simulink model "ackerman_ROS_controller_neuro_2022_v2"  (R2024b)
settings: Solver=FixedStepDiscrete  StartTime=0.0  StopTime=200  FixedStep=0.1  RelTol=1e-3
undefined symbols (not defined in the file or in its folder): Angular, Linear
libraries: neural x58, robotlib x15, robotcorelib x1
(part 2 of 2)

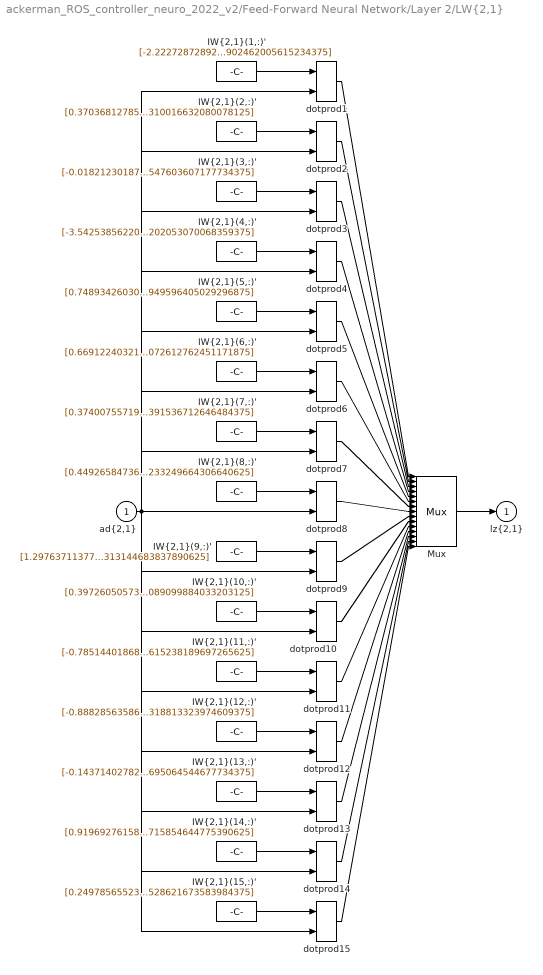
== system ackerman_ROS_controller_neuro_2022_v2/Feed-Forward Neural Network/Layer 2/LW{2,1} ==
  "ad{2,1}" : Inport  PortDimensions=30  SampleTime=0.1
      mask Display: e = 0.06;c1 = [120 230 180]/255;c2 = ([120 230 180]+0)/(256+128);c3 = ([120 230 180]+128)/(256+128);patch([0 1 1 0],[0 0 1 1],c1);patch([0 1 1 1-e 1-e 0+e],[0 0 1 1-e 0+e 0+e],c2);patch([0 0 1 1-e 0+e 0+e],[0 1 1 1-e 1-e 0+e],c3);plot([0 1 1 0 0],[0 0 1 1 0]);
  "IW{2,1}(1,:)'" : Constant  Value=[-2.222728728926282482092346981517039239406585693359375;-0.2105279558412855578364286657233606092631816864013671875;-0.172396838156845644274284268249175511300563812255859375;0.390555860841058477550546967904665507376194000244140625;0.29166384292928881905027083121240139007568359375;-0.52956405558462293914345764278550632297992706298828125;-0.2387539511607948694571490477756015025079250335693359375;-2.3297673734605712780876274337060749530792236328125;-1.0301886589615254496976604059454984962940216064453125;-0.8572014533549923154254202017909847199916839599609375;-0.96740765287111474268755273442366160452365875244140625;0.90630995398566727150324595640995539724826812744140625;-0.42554772872272794703718545861192978918552398681640625;-1.060064209881802721469057360081933438777923583984375;-0.135197213909062252668036308023147284984588623046875;0.230054241181365692892057950302842073142528533935546875;-0.827824536526168497374555954593233764171600341796875;-1.276066373600390324583031542715616524219512939453125;-0.58840911579547860998928854314726777374744415283203125;0.35688786142330453099447140630218200385570526123046875;0.795085260758974232686568939243443310260772705078125;-2.268416885537336558087417870410718023777008056640625;0.61193976284335882542819717855309136211872100830078125;1.7425116564191933665739497882896102964878082275390625;0.11927294085530919243165470788881066255271434783935546875;-0.2109230753914088374312285623091156594455242156982421875;-1.819948975500169208174838786362670361995697021484375;1.3342711728381899671802557350019924342632293701171875;1.172678912458624100878523677238263189792633056640625;-0.411449480689598467986201058010919950902462005615234375]
      mask Display: e = 0.06;c1 = [120 150 230]/255;c2 = ([120 150 230]+0)/383;c3 = ([120 150 230]+128)/383;patch([0 1 1 0],[0 0 1 1],c1);patch([0 1 1 1-e 1-e 0+e],[0 0 1 1-e 0+e 0+e],c2);patch([0 0 1 1-e 0+e 0+e],[0 1 1 1-e 1-e 0+e],c3);plot([0 1 1 0 0],[0 0 1 1 0]);disp('weights');
  "IW{2,1}(10,:)'" : Constant  Value=[0.397260505736018121325514584896154701709747314453125;-0.50051569273377294333471354548237286508083343505859375;0.02758078036917484265888589334281277842819690704345703125;0.383440619053087738965501785060041584074497222900390625;0.0314483306075712676364020126129616983234882354736328125;0.89079094780964995781147308662184514105319976806640625;-0.3737922284921084692399517734884284436702728271484375;-0.2002468106304216011182006695889867842197418212890625;0.4602876671052265056260921483044512569904327392578125;0.300424473405391356806148905889131128787994384765625;0.1539216720517649072963450862516765482723712921142578125;0.27531316556655927030305974767543375492095947265625;-1.317788466887037213126632195780985057353973388671875;-0.25114389862770158945437515285448171198368072509765625;-0.024189059746283221585816392007473041303455829620361328125;-0.2408523864701219707740165176801383495330810546875;0.08168961019016017510718796756918891333043575286865234375;-0.08534930377349826680077882201658212579786777496337890625;0.405079373978569190484222417580895125865936279296875;-3.302395281601825605122257911716587841510772705078125;-0.289408974864118817560409979705582372844219207763671875;-0.5678096913294385927883922704495489597320556640625;0.65866437262387267370655763443210162222385406494140625;-0.61601410378164789261035139134037308394908905029296875;0.1337985101975235624482962748516001738607883453369140625;-0.442241434107712050316507657043985091149806976318359375;1.4648271622279427361945636221207678318023681640625;-0.74575093210429244106052237839321605861186981201171875;-0.325176543537462225952339167633908800780773162841796875;0.47945924442098697415559627188486047089099884033203125]
      mask Display: e = 0.06;c1 = [120 150 230]/255;c2 = ([120 150 230]+0)/383;c3 = ([120 150 230]+128)/383;patch([0 1 1 0],[0 0 1 1],c1);patch([0 1 1 1-e 1-e 0+e],[0 0 1 1-e 0+e 0+e],c2);patch([0 0 1 1-e 0+e 0+e],[0 1 1 1-e 1-e 0+e],c3);plot([0 1 1 0 0],[0 0 1 1 0]);disp('weights');
  "IW{2,1}(11,:)'" : Constant  Value=[-0.7851440186858449354900812977575697004795074462890625;-0.40208723330404050333442000919603742659091949462890625;0.70730003574929212195598893231363035738468170166015625;-0.065367184060295902003900891941157169640064239501953125;-4.2920405936075400887830255669541656970977783203125;-0.523445857646462453516278401366434991359710693359375;-0.029332229217134374310571587329832254908978939056396484375;-0.171317200281045689536085774307139217853546142578125;-0.27023493407209941974400635444908402860164642333984375;-1.6651118212079636382583203157992102205753326416015625;-0.264468105797145025537275841998052783310413360595703125;0.277586538506012170390846449663513340055942535400390625;-0.03697520577241696082548827462233020924031734466552734375;-0.086749109060326456965839270196738652884960174560546875;-0.5897102236852784784559844410978257656097412109375;0.860204401837508125794329316704533994197845458984375;3.52278173836524644002565764822065830230712890625;-3.404212909954015042757191622513346374034881591796875;-2.895449655572719382945479082991369068622589111328125;-1.9360634251116242143808676701155491173267364501953125;1.0168561706644438924485029929201118648052215576171875;1.5208740618630673946398701446014456450939178466796875;1.18377350921994572985340710147283971309661865234375;0.257753028254375793348884826627909205853939056396484375;1.3769223840811586345722616897546686232089996337890625;-0.2545354697793398290883715162635780870914459228515625;0.154239895895388612334642175483168102800846099853515625;-0.435963640834392152090259742180933244526386260986328125;0.72813713755268627547678761402494274079799652099609375;0.66551241615256151451518462636158801615238189697265625]
      mask Display: e = 0.06;c1 = [120 150 230]/255;c2 = ([120 150 230]+0)/383;c3 = ([120 150 230]+128)/383;patch([0 1 1 0],[0 0 1 1],c1);patch([0 1 1 1-e 1-e 0+e],[0 0 1 1-e 0+e 0+e],c2);patch([0 0 1 1-e 0+e 0+e],[0 1 1 1-e 1-e 0+e],c3);plot([0 1 1 0 0],[0 0 1 1 0]);disp('weights');
  "IW{2,1}(12,:)'" : Constant  Value=[-0.88828563586649111893933650208055041730403900146484375;-0.6287976390637479706668955259374342858791351318359375;0.140039962452482902310890722219482995569705963134765625;0.34178216493342272741529086488299071788787841796875;0.06889275826908593247654977176352986134588718414306640625;-2.720725732529100771017738225054927170276641845703125;-1.1686144782811760389762412160052917897701263427734375;-0.04765305455937184075931867255349061451852321624755859375;0.1892635702445351342237955805103410966694355010986328125;-0.337729970142503777008613496946054510772228240966796875;0.26819643917410329603256968766800127923488616943359375;-0.073970398171442852675028234443743713200092315673828125;0.67889553499922550283685040994896553456783294677734375;0.2277097388882860229397664397765765897929668426513671875;0.17970819867203224884377732450957410037517547607421875;3.38343871560046860480497343814931809902191162109375;0.0859002580832470552518742579195532016456127166748046875;-0.365418601907997409039552394460770301520824432373046875;0.57476314636036018868026076233945786952972412109375;3.5484404227567569733992058900184929370880126953125;1.728437779847022515156140798353590071201324462890625;-0.855695122888823878071207218454219400882720947265625;1.677341944427493292124609070015139877796173095703125;0.1865942059121843410451901945634745061397552490234375;0.92489997299214277148848850629292428493499755859375;-0.64739057139335931534418477895087562501430511474609375;-1.596020893984157584810645857942290604114532470703125;0.94338078668932912052014216897077858448028564453125;1.0906949421572011971193205681629478931427001953125;-0.83878359303965088766830149324960075318813323974609375]
      mask Display: e = 0.06;c1 = [120 150 230]/255;c2 = ([120 150 230]+0)/383;c3 = ([120 150 230]+128)/383;patch([0 1 1 0],[0 0 1 1],c1);patch([0 1 1 1-e 1-e 0+e],[0 0 1 1-e 0+e 0+e],c2);patch([0 0 1 1-e 0+e 0+e],[0 1 1 1-e 1-e 0+e],c3);plot([0 1 1 0 0],[0 0 1 1 0]);disp('weights');
  "IW{2,1}(13,:)'" : Constant  Value=[-0.143714027822973544612494833927485160529613494873046875;0.44915448478707187263125888421200215816497802734375;0.376342062861311277277565068288822658360004425048828125;0.2972881796216662042553480205242522060871124267578125;-0.262879525804558422663603778346441686153411865234375;0.669912040415586940156345008290372788906097412109375;0.55179800426891001396967340042465366423130035400390625;-0.1280188538305278289630706467505660839378833770751953125;-0.26870732789751361480057312292046844959259033203125;-0.88992954257796819117487530093058012425899505615234375;0.10084960208333006159708844506894820369780063629150390625;-0.135564623109469206685417930202675051987171173095703125;0.05726056048422868693936749195927404798567295074462890625;-0.69087484836309298597001316011301241815090179443359375;-0.364074919202029223530558965649106539785861968994140625;-0.68698815425119785782470671620103530585765838623046875;-0.2989794608073983450680088935769163072109222412109375;-0.2292420658214328887947175417139078490436077117919921875;-0.45694834929996697159282348366104997694492340087890625;0.057371376318434579022476071941127884201705455780029296875;-0.00556462694212314819275366772899360512383282184600830078125;0.7850567827472574311542530267615802586078643798828125;0.25807628646158031759938467075699009001255035400390625;-0.219895909726642690973363869488821364939212799072265625;-1.6058331677712154306192360309069044888019561767578125;0.297515994915471593262878968744189478456974029541015625;-0.13003496096245992230677757106604985892772674560546875;-0.32177689840712420110691027730354107916355133056640625;0.0766703441941760377442705021167057566344738006591796875;0.68248575195410177141042140647186897695064544677734375]
      mask Display: e = 0.06;c1 = [120 150 230]/255;c2 = ([120 150 230]+0)/383;c3 = ([120 150 230]+128)/383;patch([0 1 1 0],[0 0 1 1],c1);patch([0 1 1 1-e 1-e 0+e],[0 0 1 1-e 0+e 0+e],c2);patch([0 0 1 1-e 0+e 0+e],[0 1 1 1-e 1-e 0+e],c3);plot([0 1 1 0 0],[0 0 1 1 0]);disp('weights');
  "IW{2,1}(14,:)'" : Constant  Value=[0.91969276158981216884313880655099637806415557861328125;0.01449508507313798134907845138741322443820536136627197265625;-0.024841524328765525464479679840223980136215686798095703125;0.475942644087020527710052419934072531759738922119140625;-0.66794373102359194671606701376731507480144500732421875;0.21243174640298911892699607051326893270015716552734375;-0.060849636143924780429248500013272860087454319000244140625;0.288282346155616375771302273278706707060337066650390625;0.280732424646566947057380048136110417544841766357421875;0.2220524545058630561111812085073324851691722869873046875;0.2369034334743520542332362310844473540782928466796875;-0.03729924671213581677253756652135052718222141265869140625;1.0143682463285033090727438320755027234554290771484375;-0.7815859333193930780225855414755642414093017578125;0.57258736722684455688892057878547348082065582275390625;0.35814399580322364702311688233749009668827056884765625;0.64259443013373529485221524737426079809665679931640625;-0.68301410998834699572768158759572543203830718994140625;-0.63194693767695875319390097502036951482295989990234375;-0.2370940255283547626330431512542418204247951507568359375;-0.328446483524902743678097749580047093331813812255859375;0.4236807135574398586186362081207334995269775390625;0.09468149668269500163209073662073933519423007965087890625;0.54508401115510152212806360694230534136295318603515625;0.4329377453036225009697091081761755049228668212890625;0.2318409242532646075130031704247812740504741668701171875;-0.07788041732279683826423166692620725370943546295166015625;1.732288734516942430019526000251062214374542236328125;-0.62127850580790855428148233841056935489177703857421875;-0.08755901720081916972393543119324021972715854644775390625]
      mask Display: e = 0.06;c1 = [120 150 230]/255;c2 = ([120 150 230]+0)/383;c3 = ([120 150 230]+128)/383;patch([0 1 1 0],[0 0 1 1],c1);patch([0 1 1 1-e 1-e 0+e],[0 0 1 1-e 0+e 0+e],c2);patch([0 0 1 1-e 0+e 0+e],[0 1 1 1-e 1-e 0+e],c3);plot([0 1 1 0 0],[0 0 1 1 0]);disp('weights');
  "IW{2,1}(15,:)'" : Constant  Value=[0.249785655239535053784294404977117665112018585205078125;0.73847329316424270562180254273698665201663970947265625;0.465590157117974523526271468654158525168895721435546875;-1.4664444230598145946231625202926807105541229248046875;0.09552762587386252890464533038539229892194271087646484375;-0.68536312255041187402326841038302518427371978759765625;-1.154815920318017941070820597815327346324920654296875;-0.323928699724852220409587744143209420144557952880859375;-0.370249587866944562808413365928572602570056915283203125;0.0389325824217096327917175813126959837973117828369140625;-1.993732515225736801056655167485587298870086669921875;0.04113107734049718799962391813096473924815654754638671875;-0.262819013803644363491684998734854161739349365234375;-0.473812061061643863268955101375468075275421142578125;0.132618304135100173457573191626579500734806060791015625;-1.1334068367848046943180406742612831294536590576171875;-0.6135879731176652196467102839960716664791107177734375;0.2134956515440565028018937709930469281971454620361328125;-0.1658605608926594088270434212972759269177913665771484375;-0.97371264213567132461690789568820036947727203369140625;-0.07709796244982607127393947621385450474917888641357421875;0.68597352663209665291077499205130152404308319091796875;-0.358154116190059712554472071133204735815525054931640625;0.159281117085610268713224968450958840548992156982421875;-0.2111179695429933611539041748983436264097690582275390625;0.45696544949359474419026128089171834290027618408203125;-0.757966704596435558727307579829357564449310302734375;-0.5657492883728132415654954456840641796588897705078125;-0.72239652871486137453160836230381391942501068115234375;-0.79745618550237595822949288049130700528621673583984375]
      mask Display: e = 0.06;c1 = [120 150 230]/255;c2 = ([120 150 230]+0)/383;c3 = ([120 150 230]+128)/383;patch([0 1 1 0],[0 0 1 1],c1);patch([0 1 1 1-e 1-e 0+e],[0 0 1 1-e 0+e 0+e],c2);patch([0 0 1 1-e 0+e 0+e],[0 1 1 1-e 1-e 0+e],c3);plot([0 1 1 0 0],[0 0 1 1 0]);disp('weights');
  "IW{2,1}(2,:)'" : Constant  Value=[0.37036812785328787622773916154983453452587127685546875;0.2372351393039373868010244450488244183361530303955078125;-0.08208151238239615177239016929888748563826084136962890625;-0.756141526114650464052147071924991905689239501953125;2.0086812621638596709772173198871314525604248046875;0.1690215724509795958141467053792439401149749755859375;-0.407657496635374538840324021293781697750091552734375;-0.3095937052135770972682848878321237862110137939453125;0.195510129566937196354814432197599671781063079833984375;0.5037980330495239744692526073777116835117340087890625;0.443237905161040168788844084701850078999996185302734375;-0.490943066941660510860145905098761431872844696044921875;0.70589503611337622857035967172123491764068603515625;-0.8529065119141279183168080635368824005126953125;0.055669596706750264225593838318673078902065753936767578125;0.625338821924220411574424360878765583038330078125;-1.087989422027583419350094118271954357624053955078125;1.07158158947521808812552990275435149669647216796875;1.48611353906423016013604865293018519878387451171875;0.958090545814744842800791957415640354156494140625;-0.2323317667295948518724202358498587273061275482177734375;-1.346824753200186020052342428243719041347503662109375;-0.4751862921685303664531829781481064856052398681640625;0.5088422892649340223414355932618491351604461669921875;0.94146787964793243741468131702276878058910369873046875;0.138924248447489073754468336119316518306732177734375;-0.2055196930009268729833138422691263258457183837890625;-1.209963306279714156943327907356433570384979248046875;-0.6989560104743810509120294227614067494869232177734375;0.17232859067709249689670514271710999310016632080078125]
      mask Display: e = 0.06;c1 = [120 150 230]/255;c2 = ([120 150 230]+0)/383;c3 = ([120 150 230]+128)/383;patch([0 1 1 0],[0 0 1 1],c1);patch([0 1 1 1-e 1-e 0+e],[0 0 1 1-e 0+e 0+e],c2);patch([0 0 1 1-e 0+e 0+e],[0 1 1 1-e 1-e 0+e],c3);plot([0 1 1 0 0],[0 0 1 1 0]);disp('weights');
  "IW{2,1}(3,:)'" : Constant  Value=[-0.0182123018709974167361753671912083518691360950469970703125;0.024485940403517043872927416714446735568344593048095703125;0.2128298437880238314079406336531974375247955322265625;-0.051489579338525791329939096385714947246015071868896484375;-0.31852585166436975239179218988283537328243255615234375;0.206244344898872056237593142213881947100162506103515625;-0.400235552853889287039379496491164900362491607666015625;0.3591282928342776070707031976780854165554046630859375;-0.08424416730005150621973797342434409074485301971435546875;0.58898108879171007234987200718023814260959625244140625;-0.29721325209900217867442506758379749953746795654296875;-0.362388635788180979435679773814626969397068023681640625;-0.329638246275588964184777296395623125135898590087890625;0.226923828148602513277154457682627253234386444091796875;-0.483766509869606731175650793375098146498203277587890625;0.19172010346523549184638568476657383143901824951171875;-0.0263940785096612971771801170461912988685071468353271484375;-0.0005120153139836400822682005440356078906916081905364990234375;-1.0270891419762746554766863482655026018619537353515625;0.1059209548060698613536345646934933029115200042724609375;-0.4764076619161372594390968515654094517230987548828125;-0.329461204090122639076554378334549255669116973876953125;-0.11978287653907686294285639405643451027572154998779296875;0.411122448073615365249366959687904454767704010009765625;0.130648242560915506249585860132356174290180206298828125;-0.076200560206313994182636406549136154353618621826171875;-0.007143702287312325878432250902960731764324009418487548828125;-0.409182084200852280719828968358342535793781280517578125;0.3603122929486672898491406158427707850933074951171875;-0.313453816588288469713319273068918846547603607177734375]
      mask Display: e = 0.06;c1 = [120 150 230]/255;c2 = ([120 150 230]+0)/383;c3 = ([120 150 230]+128)/383;patch([0 1 1 0],[0 0 1 1],c1);patch([0 1 1 1-e 1-e 0+e],[0 0 1 1-e 0+e 0+e],c2);patch([0 0 1 1-e 0+e 0+e],[0 1 1 1-e 1-e 0+e],c3);plot([0 1 1 0 0],[0 0 1 1 0]);disp('weights');
  "IW{2,1}(4,:)'" : Constant  Value=[-3.5425385622002547592046539648436009883880615234375;0.4922999974317985305560796405188739299774169921875;0.56569220858917323990766590213752351701259613037109375;0.25133938159345758922569302740157581865787506103515625;1.87960059681972069256516988389194011688232421875;-1.12608026029798935496728518046438694000244140625;-1.6290518269770715154010076730628497898578643798828125;-0.433087998011002561771221053277258761227130889892578125;1.1179898320468755201773092267103493213653564453125;3.37981348955477667317381929024122655391693115234375;-0.1173248613884605717760933885074337013065814971923828125;-0.91395205660366241051661972960573621094226837158203125;-0.97563873657677679940292136961943469941616058349609375;1.102527619234269451453656074590981006622314453125;-0.425011913946025166044506704565719701349735260009765625;4.15177274562676057456656053545884788036346435546875;0.340566276566583836515889061047346331179141998291015625;4.73107976353957848658637885819189250469207763671875;3.270112081000670745112302029156126081943511962890625;0.1408655540336380129762261503856279887259006500244140625;0.64206426165633267988397392400656826794147491455078125;-2.104320923987035740765350055880844593048095703125;1.455279991199464717510636546649038791656494140625;-2.114349858043695018494645410100929439067840576171875;-0.2035498565875284715520621148243662901222705841064453125;0.28110322086755845649719276480027474462985992431640625;-0.29348950925690953095426038998994044959545135498046875;-6.462763781584808242541839717887341976165771484375;-0.158628549953156561258538204128853976726531982421875;-0.77840849267862777249860073425224982202053070068359375]
      mask Display: e = 0.06;c1 = [120 150 230]/255;c2 = ([120 150 230]+0)/383;c3 = ([120 150 230]+128)/383;patch([0 1 1 0],[0 0 1 1],c1);patch([0 1 1 1-e 1-e 0+e],[0 0 1 1-e 0+e 0+e],c2);patch([0 0 1 1-e 0+e 0+e],[0 1 1 1-e 1-e 0+e],c3);plot([0 1 1 0 0],[0 0 1 1 0]);disp('weights');
  "IW{2,1}(5,:)'" : Constant  Value=[0.748934260300509802021906580193899571895599365234375;-0.260024756870508910733263974179862998425960540771484375;-0.209463383056132490533940426757908426225185394287109375;-0.00665895379365262322923779692018797504715621471405029296875;-0.57496797491057793916269247347372584044933319091796875;0.1294097822784119611316810960488510318100452423095703125;0.2238690780320813089598885881059686653316020965576171875;-0.00644720386367587071363427497772136121056973934173583984375;0.0122289871710016574690715884798919432796537876129150390625;0.53214717812383316442037539673037827014923095703125;-0.03438986009357984652279327519863727502524852752685546875;-0.276697975624961289842218548074015416204929351806640625;0.059191783604105034644060623350014793686568737030029296875;-0.60009831824530845967302639110130257904529571533203125;0.0872388227404568838974086020243703387677669525146484375;-0.4490608764886501180768618723959662020206451416015625;0.070375468096007198770536206211545504629611968994140625;0.259819826824651378682773383843596093356609344482421875;-0.4458494845662677175113230987335555255413055419921875;-0.01557199597368099340533031949007636285386979579925537109375;-0.314025829967536085352008967674919404089450836181640625;0.355495617216032788743262926800525747239589691162109375;-0.37642904997360793206695461776689626276493072509765625;-0.00842159491173539997976860149719868786633014678955078125;-0.75040971594851912929158288534381426870822906494140625;-0.740921794330680061335669961408711969852447509765625;-0.007797684022548504768901356243304689996875822544097900390625;0.71129076975495575396735148387961089611053466796875;0.31132072686855660759164265982690267264842987060546875;0.7242296877328360249492789080250076949596405029296875]
      mask Display: e = 0.06;c1 = [120 150 230]/255;c2 = ([120 150 230]+0)/383;c3 = ([120 150 230]+128)/383;patch([0 1 1 0],[0 0 1 1],c1);patch([0 1 1 1-e 1-e 0+e],[0 0 1 1-e 0+e 0+e],c2);patch([0 0 1 1-e 0+e 0+e],[0 1 1 1-e 1-e 0+e],c3);plot([0 1 1 0 0],[0 0 1 1 0]);disp('weights');
  "IW{2,1}(6,:)'" : Constant  Value=[0.6691224032183182846011959554743953049182891845703125;-0.077899016506656926228657766841934062540531158447265625;-0.02977319013924108193069884009673842228949069976806640625;0.516275449996285384912653171340934932231903076171875;0.065904792188196281710332868897239677608013153076171875;1.1827724732815070307623273038188926875591278076171875;-0.7921366599845403033697266437229700386524200439453125;-1.4722908061548418690023254384868778288364410400390625;0.10956457541477628014892076180331059731543064117431640625;-0.0493860379286160944278805118301534093916416168212890625;-1.236851433593874727279171565896831452846527099609375;0.328506720181672429159647208507522009313106536865234375;-0.8714775076422360822192558771348558366298675537109375;-0.05116444042981006801174004294807673431932926177978515625;0.454327646038264310046628224881715141236782073974609375;-0.71114867816480098472453619251609779894351959228515625;-0.03490230386603428158753814614101429469883441925048828125;-0.28786005960766514188975406796089373528957366943359375;0.230842452883788962214595130717498250305652618408203125;0.168030368301299137812065964681096374988555908203125;-0.294740061534179365043684128977474756538867950439453125;-0.86302757987221123681109702374669723212718963623046875;-0.54941718152965013377553304962930269539356231689453125;0.220925404586086837621650147411855868995189666748046875;-1.3594204163210752422941141048795543611049652099609375;-0.53886101528822727413370330395991913974285125732421875;-0.396998483925780021319695833881269209086894989013671875;-0.464034534801797293734892946304171346127986907958984375;-0.45253068075537716818956823772168718278408050537109375;0.42311102353099883099929456875543110072612762451171875]
      mask Display: e = 0.06;c1 = [120 150 230]/255;c2 = ([120 150 230]+0)/383;c3 = ([120 150 230]+128)/383;patch([0 1 1 0],[0 0 1 1],c1);patch([0 1 1 1-e 1-e 0+e],[0 0 1 1-e 0+e 0+e],c2);patch([0 0 1 1-e 0+e 0+e],[0 1 1 1-e 1-e 0+e],c3);plot([0 1 1 0 0],[0 0 1 1 0]);disp('weights');
  "IW{2,1}(7,:)'" : Constant  Value=[0.374007557198554663191458757864893414080142974853515625;0.186719102458715202619288220375892706215381622314453125;-0.372357642079240658272709652010235004127025604248046875;-0.2236629281337665642315215563940000720322132110595703125;-0.52666750684419605388342233709408901631832122802734375;-0.00180119958290875215554949217988678356050513684749603271484375;0.06569587491566621084704280519872554577887058258056640625;0.91245199976357505011748116885428316891193389892578125;0.2173329965744563441187864327730494551360607147216796875;-0.316977260964661888831273017785861156880855560302734375;0.08763923658341753186729050639769411645829677581787109375;-0.2443741874984831363715187535490258596837520599365234375;0.0966798716890060749751256707895663566887378692626953125;-0.2969270463070332599642142668017186224460601806640625;0.05953626015160069784304397444429923780262470245361328125;-0.410383712678033696352741799273644573986530303955078125;-0.1473310748515783419332336734441923908889293670654296875;-0.337855064877262412093017474035150371491909027099609375;-0.5199197307999867678773853185703046619892120361328125;0.27224215422965880595285170784336514770984649658203125;-0.5048217645343242576672082577715627849102020263671875;-0.133341236434949717004627700589480809867382049560546875;0.1494982005733958008164563580066896975040435791015625;0.037345581409195145738966203907693852670490741729736328125;-0.1648933128849285056904960811152704991400241851806640625;-0.5752399248438841983244174116407521069049835205078125;-0.259617862943391786156865919110714457929134368896484375;0.63016515402819905933284871935029514133930206298828125;-0.292702356986898226676174772364902310073375701904296875;-0.4258597860960990910683676702319644391536712646484375]
      mask Display: e = 0.06;c1 = [120 150 230]/255;c2 = ([120 150 230]+0)/383;c3 = ([120 150 230]+128)/383;patch([0 1 1 0],[0 0 1 1],c1);patch([0 1 1 1-e 1-e 0+e],[0 0 1 1-e 0+e 0+e],c2);patch([0 0 1 1-e 0+e 0+e],[0 1 1 1-e 1-e 0+e],c3);plot([0 1 1 0 0],[0 0 1 1 0]);disp('weights');
  "IW{2,1}(8,:)'" : Constant  Value=[0.449265847363149617432753757384489290416240692138671875;0.55400761460902081534385388295049779117107391357421875;0.198967673109008258425234316746355034410953521728515625;-0.116864141677579080891291596344672143459320068359375;-0.51715852792536864956929321124334819614887237548828125;-0.17326883447011187655562025611288845539093017578125;-0.2108875108098115236376912662308313883841037750244140625;-0.518438291201025247545430829632095992565155029296875;0.10336210404818668706639073207043111324310302734375;-0.94300234486291334423668786257621832191944122314453125;0.1631418722011565847207492652159999124705791473388671875;0.52238458095239626022276979711023159325122833251953125;-0.670860669847113566532925688079558312892913818359375;0.2380314157178698708516861870521097443997859954833984375;0.04794803337682269905872800563884084112942218780517578125;0.2389001860912173536011238184073590673506259918212890625;0.130821538950658011746241982109495438635349273681640625;-0.62061651165405062879898423489066772162914276123046875;-0.90093267331892945559701502133975736796855926513671875;0.0330097545095187905328515398650779388844966888427734375;0.103376264560557540317375924132647924125194549560546875;-0.6561096676197710753086766999331302940845489501953125;-0.1687930692497993934164668416997301392257213592529296875;0.40843068153392392272138522457680664956569671630859375;-0.494354870784107502945659007309586741030216217041015625;-0.00065137746861309610280077464494752348400652408599853515625;-0.326592212939607218213922124050441198050975799560546875;0.5675560047158600962546870505320839583873748779296875;0.159509134799981355801179461195715703070163726806640625;0.336688387109719489131975933560170233249664306640625]
      mask Display: e = 0.06;c1 = [120 150 230]/255;c2 = ([120 150 230]+0)/383;c3 = ([120 150 230]+128)/383;patch([0 1 1 0],[0 0 1 1],c1);patch([0 1 1 1-e 1-e 0+e],[0 0 1 1-e 0+e 0+e],c2);patch([0 0 1 1-e 0+e 0+e],[0 1 1 1-e 1-e 0+e],c3);plot([0 1 1 0 0],[0 0 1 1 0]);disp('weights');
  "IW{2,1}(9,:)'" : Constant  Value=[1.2976371137701765423599908899632282555103302001953125;0.1828995024746147002314700102942879311740398406982421875;-0.1459844870837760655302162149382638745009899139404296875;-0.7716347832951153673519684161874465644359588623046875;-1.008587595844738782346894367947243154048919677734375;0.72572420654990843491560781330917961895465850830078125;0.578550443260642310860930592752993106842041015625;1.0738987820404102269122859070193953812122344970703125;0.366361614746913255569182865656330250203609466552734375;0.11811333747112799652523307258888962678611278533935546875;-0.275218061708887073990581484395079314708709716796875;-0.42445845546834160000315705474349670112133026123046875;1.8080563236297262363905247184447944164276123046875;0.76585686721014012423580652466625906527042388916015625;0.3584041608410906132320405959035269916057586669921875;0.190444569370965377519411276807659305632114410400390625;0.3302942978489229464145182646461762487888336181640625;0.1443874498570860420709749405432376079261302947998046875;0.099271530912751926312154182596714235842227935791015625;-0.9249896991418558034325769767747260630130767822265625;-1.6136715319944270330410063252202235162258148193359375;4.47481788656067980269881445565260946750640869140625;-1.1959973670495134268065839933115057647228240966796875;-0.10755063581194811150876233796225278638303279876708984375;1.4901771068724392055315774996415711939334869384765625;0.2347105260598317533204948404090828262269496917724609375;1.9622605255737732843357434830977581441402435302734375;1.1035114222626660751558347328682430088520050048828125;-0.73184666714602553128088402445428073406219482421875;-1.161733468839637684055787758552469313144683837890625]
      mask Display: e = 0.06;c1 = [120 150 230]/255;c2 = ([120 150 230]+0)/383;c3 = ([120 150 230]+128)/383;patch([0 1 1 0],[0 0 1 1],c1);patch([0 1 1 1-e 1-e 0+e],[0 0 1 1-e 0+e 0+e],c2);patch([0 0 1 1-e 0+e 0+e],[0 1 1 1-e 1-e 0+e],c3);plot([0 1 1 0 0],[0 0 1 1 0]);disp('weights');
  Mux : Mux  Inputs=15
      mask Display: e = 0.06;c1 = [120 150 230]/255;c2 = ([120 150 230]+0)/383;c3 = ([120 150 230]+128)/383;patch([0 1 1 0],[0 0 1 1],c1);patch([0 1 1 1-e 1-e 0+e],[0 0 1 1-e 0+e 0+e],c2);patch([0 0 1 1-e 0+e 0+e],[0 1 1 1-e 1-e 0+e],c3);plot([0 1 1 0 0],[0 0 1 1 0]);disp('Mux');
  dotprod{1..15} (15 alike) : neural/Weight Functions/dotprod
  "lz{2,1}" : Outport
      mask Display: e = 0.06;c1 = [120 230 180]/255;c2 = ([120 230 180]+0)/(256+128);c3 = ([120 230 180]+128)/(256+128);patch([0 1 1 0],[0 0 1 1],c1);patch([0 1 1 1-e 1-e 0+e],[0 0 1 1-e 0+e 0+e],c2);patch([0 0 1 1-e 0+e 0+e],[0 1 1 1-e 1-e 0+e],c3);plot([0 1 1 0 0],[0 0 1 1 0]);
  wires:
  "IW{2,1}(1,:)'"/1 -> dotprod1/1
  "ad{2,1}"/1 -> dotprod1/2, dotprod2/2, dotprod3/2, dotprod4/2, dotprod5/2, dotprod6/2, dotprod7/2, dotprod8/2, dotprod9/2, dotprod10/2, dotprod11/2, dotprod12/2, dotprod13/2, dotprod14/2, dotprod15/2
  dotprod1/1 -> Mux/1
  "IW{2,1}(2,:)'"/1 -> dotprod2/1
  dotprod2/1 -> Mux/2
  "IW{2,1}(3,:)'"/1 -> dotprod3/1
  dotprod3/1 -> Mux/3
  "IW{2,1}(4,:)'"/1 -> dotprod4/1
  dotprod4/1 -> Mux/4
  "IW{2,1}(5,:)'"/1 -> dotprod5/1
  dotprod5/1 -> Mux/5
  "IW{2,1}(6,:)'"/1 -> dotprod6/1
  dotprod6/1 -> Mux/6
  "IW{2,1}(7,:)'"/1 -> dotprod7/1
  dotprod7/1 -> Mux/7
  "IW{2,1}(8,:)'"/1 -> dotprod8/1
  dotprod8/1 -> Mux/8
  "IW{2,1}(9,:)'"/1 -> dotprod9/1
  dotprod9/1 -> Mux/9
  "IW{2,1}(10,:)'"/1 -> dotprod10/1
  dotprod10/1 -> Mux/10
  "IW{2,1}(11,:)'"/1 -> dotprod11/1
  dotprod11/1 -> Mux/11
  "IW{2,1}(12,:)'"/1 -> dotprod12/1
  dotprod12/1 -> Mux/12
  "IW{2,1}(13,:)'"/1 -> dotprod13/1
  dotprod13/1 -> Mux/13
  "IW{2,1}(14,:)'"/1 -> dotprod14/1
  dotprod14/1 -> Mux/14
  "IW{2,1}(15,:)'"/1 -> dotprod15/1
  dotprod15/1 -> Mux/15
  Mux/1 -> "lz{2,1}"/1

== system ackerman_ROS_controller_neuro_2022_v2/Feed-Forward Neural Network/Layer 3/Delays 1 ==
  "p{3}" : Inport  PortDimensions=15  SampleTime=0.1
      mask Display: e = 0.06;c1 = [120 230 180]/255;c2 = ([120 230 180]+0)/(256+128);c3 = ([120 230 180]+128)/(256+128);patch([0 1 1 0],[0 0 1 1],c1);patch([0 1 1 1-e 1-e 0+e],[0 0 1 1-e 0+e 0+e],c2);patch([0 0 1 1-e 0+e 0+e],[0 1 1 1-e 1-e 0+e],c3);plot([0 1 1 0 0],[0 0 1 1 0]);
  mux : Mux  Inputs=1
      mask Display: e = 0.06;c1 = [120 150 230]/255;c2 = ([120 150 230]+0)/383;c3 = ([120 150 230]+128)/383;patch([0 1 1 0],[0 0 1 1],c1);patch([0 1 1 1-e 1-e 0+e],[0 0 1 1-e 0+e 0+e],c2);patch([0 0 1 1-e 0+e 0+e],[0 1 1 1-e 1-e 0+e],c3);plot([0 1 1 0 0],[0 0 1 1 0]);disp('Mux')
  "pd{3,2}" : Outport
      mask Display: e = 0.06;c1 = [120 230 180]/255;c2 = ([120 230 180]+0)/(256+128);c3 = ([120 230 180]+128)/(256+128);patch([0 1 1 0],[0 0 1 1],c1);patch([0 1 1 1-e 1-e 0+e],[0 0 1 1-e 0+e 0+e],c2);patch([0 0 1 1-e 0+e 0+e],[0 1 1 1-e 1-e 0+e],c3);plot([0 1 1 0 0],[0 0 1 1 0]);
  wires:
  "p{3}"/1 -> mux/1
  mux/1 -> "pd{3,2}"/1

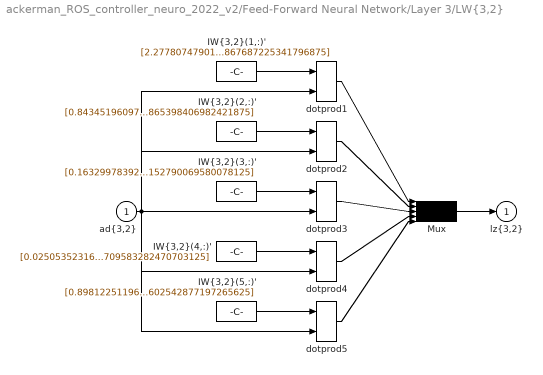
== system ackerman_ROS_controller_neuro_2022_v2/Feed-Forward Neural Network/Layer 3/LW{3,2} ==
  "ad{3,2}" : Inport  PortDimensions=15  SampleTime=0.1
      mask Display: e = 0.06;c1 = [120 230 180]/255;c2 = ([120 230 180]+0)/(256+128);c3 = ([120 230 180]+128)/(256+128);patch([0 1 1 0],[0 0 1 1],c1);patch([0 1 1 1-e 1-e 0+e],[0 0 1 1-e 0+e 0+e],c2);patch([0 0 1 1-e 0+e 0+e],[0 1 1 1-e 1-e 0+e],c3);plot([0 1 1 0 0],[0 0 1 1 0]);
  "IW{3,2}(1,:)'" : Constant  Value=[2.2778074790171043417785767815075814723968505859375;0.461364223239852655478188125925953499972820281982421875;-0.4438798918756721167966361463186331093311309814453125;-0.029440838981192492262994875318327103741466999053955078125;2.94234702403731152031696183257736265659332275390625;-0.65283796921311132432919066559406928718090057373046875;1.833125740660989766439570303191430866718292236328125;1.0540729383719382727946367594995535910129547119140625;-0.53727115747822218327911514279549010097980499267578125;0.7398954846553513764462195467785932123661041259765625;-4.35067109267328699928611968061886727809906005859375;-4.56656549351669927006014404469169676303863525390625;-0.26998174782680006700275043840520083904266357421875;0.7316173511890216030195688290405087172985076904296875;-1.3049081564867310856214999148505739867687225341796875]
      mask Display: e = 0.06;c1 = [120 150 230]/255;c2 = ([120 150 230]+0)/383;c3 = ([120 150 230]+128)/383;patch([0 1 1 0],[0 0 1 1],c1);patch([0 1 1 1-e 1-e 0+e],[0 0 1 1-e 0+e 0+e],c2);patch([0 0 1 1-e 0+e 0+e],[0 1 1 1-e 1-e 0+e],c3);plot([0 1 1 0 0],[0 0 1 1 0]);disp('weights');
  "IW{3,2}(2,:)'" : Constant  Value=[0.843451960972080971856712494627572596073150634765625;0.889155726094772003165189744322560727596282958984375;-0.276334761543234164182791801067651249468326568603515625;2.05706428394446305674136965535581111907958984375;-0.015874437000282230758596568875873344950377941131591796875;0.620133986387136015849819159484468400478363037109375;1.01199276940510429767527966760098934173583984375;-0.58917144627627637820665995604940690100193023681640625;0.084406544047432918720375027987756766378879547119140625;-0.178129129125695839785947782729635946452617645263671875;0.25074402397468198433472252872888930141925811767578125;2.50966939491780660631548016681335866451263427734375;-1.1501822614900110153257628553546965122222900390625;-0.980585266442811853693228840711526572704315185546875;-0.291151578733516991359664416449959389865398406982421875]
      mask Display: e = 0.06;c1 = [120 150 230]/255;c2 = ([120 150 230]+0)/383;c3 = ([120 150 230]+128)/383;patch([0 1 1 0],[0 0 1 1],c1);patch([0 1 1 1-e 1-e 0+e],[0 0 1 1-e 0+e 0+e],c2);patch([0 0 1 1-e 0+e 0+e],[0 1 1 1-e 1-e 0+e],c3);plot([0 1 1 0 0],[0 0 1 1 0]);disp('weights');
  "IW{3,2}(3,:)'" : Constant  Value=[0.163299783926757147156649807584472000598907470703125;0.09305778235220445171460568190013873390853404998779296875;1.0539247057268184004641398132662288844585418701171875;1.6666638173833818736824241568683646619319915771484375;-1.0431128469984598527986463523120619356632232666015625;-0.666180568877114520631721461541019380092620849609375;-1.5297983685734235503872469053021632134914398193359375;1.02358352875155755867808693437837064266204833984375;2.33400624594746464168792954296804964542388916015625;-0.51952559031888168039614583904040046036243438720703125;2.62189990769854741614608428790234029293060302734375;0.925985768123850139232899891794659197330474853515625;0.60263518725551168397913670560228638350963592529296875;0.2029748329091563274761966795267653651535511016845703125;0.66465799329676678031120218292926438152790069580078125]
      mask Display: e = 0.06;c1 = [120 150 230]/255;c2 = ([120 150 230]+0)/383;c3 = ([120 150 230]+128)/383;patch([0 1 1 0],[0 0 1 1],c1);patch([0 1 1 1-e 1-e 0+e],[0 0 1 1-e 0+e 0+e],c2);patch([0 0 1 1-e 0+e 0+e],[0 1 1 1-e 1-e 0+e],c3);plot([0 1 1 0 0],[0 0 1 1 0]);disp('weights');
  "IW{3,2}(4,:)'" : Constant  Value=[0.0250535231699762876711456982548043015412986278533935546875;0.9532050743652862312416118584224022924900054931640625;-1.849786896597151564236582999001257121562957763671875;5.5108841046447398781538140610791742801666259765625;-1.50469263226082805573469158844090998172760009765625;2.11345005489201920312325455597601830959320068359375;-0.6029408695746401036785755422897636890411376953125;-2.3474978761465354892834511701948940753936767578125;1.15546436537457264392969591426663100719451904296875;-0.2213756904819754456337221881767618469893932342529296875;-1.154717800599419863516459372476674616336822509765625;3.05245229879936896821845948579721152782440185546875;-0.97233184742671741052078004940995015203952789306640625;1.00339581658149423759596174932084977626800537109375;-0.59323278075888563609652237573754973709583282470703125]
      mask Display: e = 0.06;c1 = [120 150 230]/255;c2 = ([120 150 230]+0)/383;c3 = ([120 150 230]+128)/383;patch([0 1 1 0],[0 0 1 1],c1);patch([0 1 1 1-e 1-e 0+e],[0 0 1 1-e 0+e 0+e],c2);patch([0 0 1 1-e 0+e 0+e],[0 1 1 1-e 1-e 0+e],c3);plot([0 1 1 0 0],[0 0 1 1 0]);disp('weights');
  "IW{3,2}(5,:)'" : Constant  Value=[0.89812251196532455477239409447065554559230804443359375;-1.734683227129370397534557923790998756885528564453125;-0.7724417488455650460110746280406601727008819580078125;-0.0612746518385229033132333142930292524397373199462890625;-0.851210555322980066961235934286378324031829833984375;-0.6380256559514843051061916412436403334140777587890625;0.3700745362683945938186980129103176295757293701171875;0.814454488378295149431096433545462787151336669921875;-0.31195861688284065582621451540035195648670196533203125;-0.473702779672403540001113242396968416869640350341796875;-1.39965818068148717401300018536858260631561279296875;-0.08080681732176613063511894097246113233268260955810546875;0.0881002050231377842326452309862361289560794830322265625;-1.3978311589065872677650759214884601533412933349609375;1.0249704447485417091456838534213602542877197265625]
      mask Display: e = 0.06;c1 = [120 150 230]/255;c2 = ([120 150 230]+0)/383;c3 = ([120 150 230]+128)/383;patch([0 1 1 0],[0 0 1 1],c1);patch([0 1 1 1-e 1-e 0+e],[0 0 1 1-e 0+e 0+e],c2);patch([0 0 1 1-e 0+e 0+e],[0 1 1 1-e 1-e 0+e],c3);plot([0 1 1 0 0],[0 0 1 1 0]);disp('weights');
  Mux : Mux  Inputs=5
      mask Display: e = 0.06;c1 = [120 150 230]/255;c2 = ([120 150 230]+0)/383;c3 = ([120 150 230]+128)/383;patch([0 1 1 0],[0 0 1 1],c1);patch([0 1 1 1-e 1-e 0+e],[0 0 1 1-e 0+e 0+e],c2);patch([0 0 1 1-e 0+e 0+e],[0 1 1 1-e 1-e 0+e],c3);plot([0 1 1 0 0],[0 0 1 1 0]);disp('Mux');
  dotprod{1..5} (5 alike) : neural/Weight Functions/dotprod
  "lz{3,2}" : Outport
      mask Display: e = 0.06;c1 = [120 230 180]/255;c2 = ([120 230 180]+0)/(256+128);c3 = ([120 230 180]+128)/(256+128);patch([0 1 1 0],[0 0 1 1],c1);patch([0 1 1 1-e 1-e 0+e],[0 0 1 1-e 0+e 0+e],c2);patch([0 0 1 1-e 0+e 0+e],[0 1 1 1-e 1-e 0+e],c3);plot([0 1 1 0 0],[0 0 1 1 0]);
  wires:
  "IW{3,2}(1,:)'"/1 -> dotprod1/1
  "ad{3,2}"/1 -> dotprod1/2, dotprod2/2, dotprod3/2, dotprod4/2, dotprod5/2
  dotprod1/1 -> Mux/1
  "IW{3,2}(2,:)'"/1 -> dotprod2/1
  dotprod2/1 -> Mux/2
  "IW{3,2}(3,:)'"/1 -> dotprod3/1
  dotprod3/1 -> Mux/3
  "IW{3,2}(4,:)'"/1 -> dotprod4/1
  dotprod4/1 -> Mux/4
  "IW{3,2}(5,:)'"/1 -> dotprod5/1
  dotprod5/1 -> Mux/5
  Mux/1 -> "lz{3,2}"/1

== system ackerman_ROS_controller_neuro_2022_v2/Feed-Forward Neural Network/Layer 4/Delays 1 ==
  "p{4}" : Inport  PortDimensions=5  SampleTime=0.1
      mask Display: e = 0.06;c1 = [120 230 180]/255;c2 = ([120 230 180]+0)/(256+128);c3 = ([120 230 180]+128)/(256+128);patch([0 1 1 0],[0 0 1 1],c1);patch([0 1 1 1-e 1-e 0+e],[0 0 1 1-e 0+e 0+e],c2);patch([0 0 1 1-e 0+e 0+e],[0 1 1 1-e 1-e 0+e],c3);plot([0 1 1 0 0],[0 0 1 1 0]);
  mux : Mux  Inputs=1
      mask Display: e = 0.06;c1 = [120 150 230]/255;c2 = ([120 150 230]+0)/383;c3 = ([120 150 230]+128)/383;patch([0 1 1 0],[0 0 1 1],c1);patch([0 1 1 1-e 1-e 0+e],[0 0 1 1-e 0+e 0+e],c2);patch([0 0 1 1-e 0+e 0+e],[0 1 1 1-e 1-e 0+e],c3);plot([0 1 1 0 0],[0 0 1 1 0]);disp('Mux')
  "pd{4,3}" : Outport
      mask Display: e = 0.06;c1 = [120 230 180]/255;c2 = ([120 230 180]+0)/(256+128);c3 = ([120 230 180]+128)/(256+128);patch([0 1 1 0],[0 0 1 1],c1);patch([0 1 1 1-e 1-e 0+e],[0 0 1 1-e 0+e 0+e],c2);patch([0 0 1 1-e 0+e 0+e],[0 1 1 1-e 1-e 0+e],c3);plot([0 1 1 0 0],[0 0 1 1 0]);
  wires:
  "p{4}"/1 -> mux/1
  mux/1 -> "pd{4,3}"/1

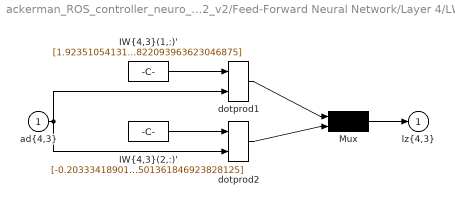
== system ackerman_ROS_controller_neuro_2022_v2/Feed-Forward Neural Network/Layer 4/LW{4,3} ==
  "ad{4,3}" : Inport  PortDimensions=5  SampleTime=0.1
      mask Display: e = 0.06;c1 = [120 230 180]/255;c2 = ([120 230 180]+0)/(256+128);c3 = ([120 230 180]+128)/(256+128);patch([0 1 1 0],[0 0 1 1],c1);patch([0 1 1 1-e 1-e 0+e],[0 0 1 1-e 0+e 0+e],c2);patch([0 0 1 1-e 0+e 0+e],[0 1 1 1-e 1-e 0+e],c3);plot([0 1 1 0 0],[0 0 1 1 0]);
  "IW{4,3}(1,:)'" : Constant  Value=[1.9235105413106616811802496158634312450885772705078125;-3.8555290721645700813269286300055682659149169921875;1.776049477637690277020965368137694895267486572265625;3.8571725327211279221728545962832868099212646484375;-0.0026154083718876279529563788628365728072822093963623046875]
      mask Display: e = 0.06;c1 = [120 150 230]/255;c2 = ([120 150 230]+0)/383;c3 = ([120 150 230]+128)/383;patch([0 1 1 0],[0 0 1 1],c1);patch([0 1 1 1-e 1-e 0+e],[0 0 1 1-e 0+e 0+e],c2);patch([0 0 1 1-e 0+e 0+e],[0 1 1 1-e 1-e 0+e],c3);plot([0 1 1 0 0],[0 0 1 1 0]);disp('weights');
  "IW{4,3}(2,:)'" : Constant  Value=[-0.2033341890117660033521218565510935150086879730224609375;0.074521261303289343391753618561779148876667022705078125;-0.255901534827980337016839484931551851332187652587890625;-0.5575334761196988342391023252275772392749786376953125;-0.83297048673436890897647799647529609501361846923828125]
      mask Display: e = 0.06;c1 = [120 150 230]/255;c2 = ([120 150 230]+0)/383;c3 = ([120 150 230]+128)/383;patch([0 1 1 0],[0 0 1 1],c1);patch([0 1 1 1-e 1-e 0+e],[0 0 1 1-e 0+e 0+e],c2);patch([0 0 1 1-e 0+e 0+e],[0 1 1 1-e 1-e 0+e],c3);plot([0 1 1 0 0],[0 0 1 1 0]);disp('weights');
  Mux : Mux  Inputs=2
      mask Display: e = 0.06;c1 = [120 150 230]/255;c2 = ([120 150 230]+0)/383;c3 = ([120 150 230]+128)/383;patch([0 1 1 0],[0 0 1 1],c1);patch([0 1 1 1-e 1-e 0+e],[0 0 1 1-e 0+e 0+e],c2);patch([0 0 1 1-e 0+e 0+e],[0 1 1 1-e 1-e 0+e],c3);plot([0 1 1 0 0],[0 0 1 1 0]);disp('Mux');
  dotprod1 : neural/Weight Functions/dotprod
  dotprod2 : neural/Weight Functions/dotprod
  "lz{4,3}" : Outport
      mask Display: e = 0.06;c1 = [120 230 180]/255;c2 = ([120 230 180]+0)/(256+128);c3 = ([120 230 180]+128)/(256+128);patch([0 1 1 0],[0 0 1 1],c1);patch([0 1 1 1-e 1-e 0+e],[0 0 1 1-e 0+e 0+e],c2);patch([0 0 1 1-e 0+e 0+e],[0 1 1 1-e 1-e 0+e],c3);plot([0 1 1 0 0],[0 0 1 1 0]);
  wires:
  "IW{4,3}(1,:)'"/1 -> dotprod1/1
  "ad{4,3}"/1 -> dotprod1/2, dotprod2/2
  dotprod1/1 -> Mux/1
  "IW{4,3}(2,:)'"/1 -> dotprod2/1
  dotprod2/1 -> Mux/2
  Mux/1 -> "lz{4,3}"/1

== matlab function ackerman_ROS_controller_neuro_2022_v2/ROS Robot/Conversion_diff_ackerman ==
  data: steering_wheel_angle input; V output; linear_vel_ackerman_kmh input; W output
function [V,W] = fcn(steering_wheel_angle, linear_vel_ackerman_kmh)

    %Aproximacion de angulo volante y velocidad linal a vel_linar y angular.
    % *************************************
    
    min_turning_radius_vehicle = 2;  % radio de giro del vehiculo. Radio minimo en el que gira 180 grados. 
    max_turning_radius_vehicle = 34; % radio de giro del vehiculo. Radio máximo con el volante girado 1º
    max_steering_wheel_angle = 90;  % angulo máximo de volante permitido (grados).
    max_vehicle_linear_speed = 50;  % velocidad máxima de vehiculo (km/h).
    
    
    % Filtrado des los valores máximos
    
    if steering_wheel_angle > max_steering_wheel_angle
        steering_wheel_angle = max_steering_wheel_angle;  
    end
    
    if steering_wheel_angle < (-1*max_steering_wheel_angle)
        steering_wheel_angle = max_steering_wheel_angle;  
    end
    
    if linear_vel_ackerman_kmh > max_vehicle_linear_speed
        linear_vel_ackerman_kmh = max_vehicle_linear_speed;
    end
    
    
    %Conversion a m/s
    linear_vel_ackerman_ms = linear_vel_ackerman_kmh/3.6; %(m/s)
    
    %Conversion a linear and angular velocity for the simulator.
    % v=rω --> ω = v/r
    
    % max_steering_wheel_angle -- > min_turning_radius_vehicle
    % steering_wheel_angle = 0 --> angular_vel_vehicle = 0;
    
    turning_radius = (max_turning_radius_vehicle-((max_turning_radius_vehicle-min_turning_radius_vehicle)/max_steering_wheel_angle)*abs(steering_wheel_angle));
    
    if steering_wheel_angle > 0
            turning_radius = turning_radius;
    elseif steering_wheel_angle < 0
            turning_radius = -1*turning_radius;
    end
    
    if abs(steering_wheel_angle) < 0.01
        angular_vel_vehicle = 0;
    else
        angular_vel_vehicle = linear_vel_ackerman_ms / turning_radius;
    end
    
    %Sin velocidad linear, tampoco debe girar
    
    if linear_vel_ackerman_ms == 0
        angular_vel_vehicle = 0;
    end
    
    
    %Rellenamos los campos del mensaje V y W
    V= linear_vel_ackerman_ms;

    W=angular_vel_vehicle;
    
    
    %********************************************************

== matlab function ackerman_ROS_controller_neuro_2022_v2/ROS Robot/MATLAB Function ==
  data: u input; y output
function y = fcn(u)
u(isinf(u))=15.0;
y = u;

== matlab function ackerman_ROS_controller_neuro_2022_v2/MATLAB Function ==
  data: stop_flag input; vel output; vel input; steering_wheel input; steering_wheel output
function [vel, steering_wheel]= stop(stop_flag,vel,steering_wheel)
    if stop_flag 
        steering_wheel=0;
        vel=0;
    else
        vel=vel;
        steering_wheel=steering_wheel;
    end

== matlab function ackerman_ROS_controller_neuro_2022_v2/Evaluacion_maniobra/evaluacion_fin ==
  data: clock input; x input; y input; theta input; stop_flag output
function stop_flag = evaluacion_fin(clock, x, y, theta)
    if x > 59 && x < 60
        if y < 4
            stop_flag = 1;
        else 
            stop_flag = 0;
        end
        else
            stop_flag = 0;
    end
end
